simulink model "HW4_2a_gradient_discrete_time_proj_bad"  (R2023b)
settings: Solver=VariableStepAuto  StartTime=0.0  StopTime=700  RelTol=1e-3
model workspace (MAT data in the model file):
  M = Simulink.Parameter
  M.Value = 0.5
  M.DataType = 'auto'
  M.Complexity = 'real'
  M.Dimensions = [1 1]
  alpha = Simulink.Parameter
  alpha.Value = 1
  alpha.DataType = 'auto'
  alpha.Complexity = 'real'
  alpha.Dimensions = [1 1]
  b = Simulink.Parameter
  b.Value = 0.1
  b.DataType = 'auto'
  b.Complexity = 'real'
  b.Dimensions = [1 1]
  k = Simulink.Parameter
  k.Value = 5
  k.DataType = 'auto'
  k.Complexity = 'real'
  k.Dimensions = [1 1]
  m = Simulink.Parameter
  m.Value = 20
  m.DataType = 'auto'
  m.Complexity = 'real'
  m.Dimensions = [1 1]
  minv = Simulink.Parameter
  minv.Value = 1
  minv.Description = 'This is written by the parameter writer block.
    | Unfortunately it needs a placeholder value, so just choosing that as 1.'
  minv.DataType = 'auto'
  minv.Complexity = 'real'
  minv.Dimensions = [1 1]
undefined symbols (not defined in the file): DiscIntNeverNeededParam
libraries: matrix_library x3
settings Model: Creator=kaleb  LastModifiedBy=kaleb

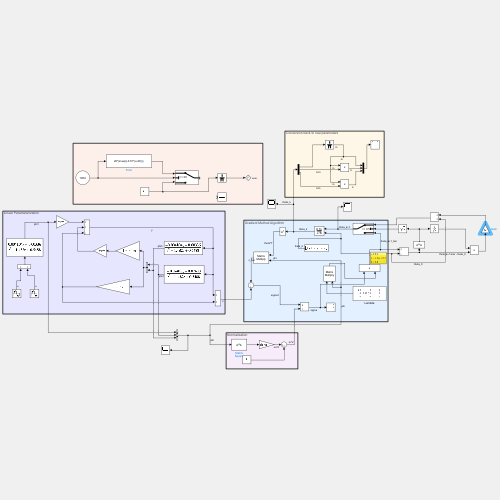
[thumbnail: Simulink's stored preview of the top-level diagram]
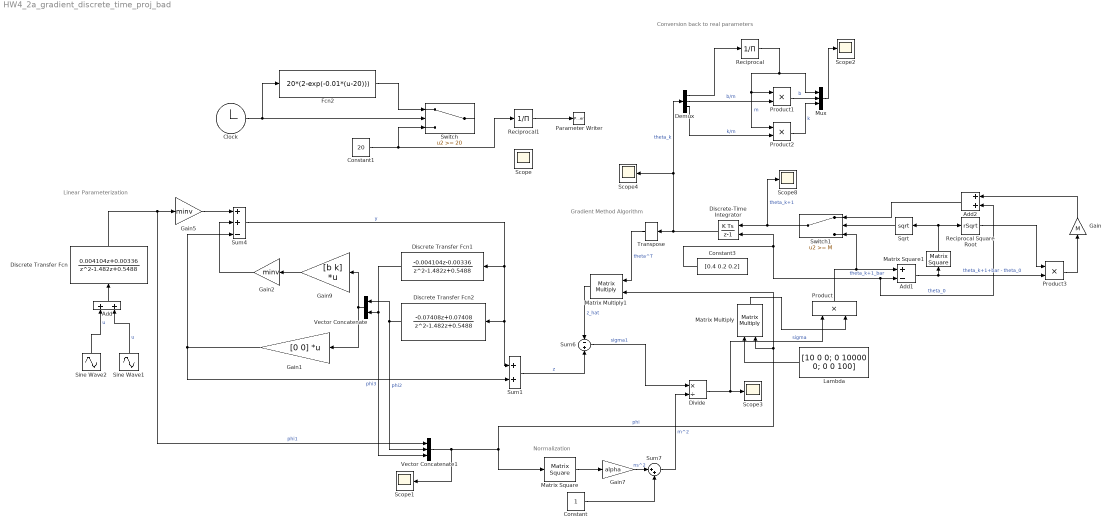
== system HW4_2a_gradient_discrete_time_proj_bad ==
  note: Gradient Method Algorithm
  note: Conversion back to real parameters
  note: Normalization
  note: Linear Parameterization
  Add : Sum
  Add1 : Sum  Inputs=+-
  Add2 : Sum
  Clock : Clock
  Constant : Constant
  Constant1 : Constant  Value=20
  Constant3 : Constant  Value=[0.4 0.2 0.2]
  Demux : Demux  Outputs=3
  Discrete Transfer Fcn : DiscreteTransferFcn  Numerator=[0.004104 0.00336]  Denominator=[1 -1.482 0.5488]
  Discrete Transfer Fcn1 : DiscreteTransferFcn  Numerator=[-0.004104 -0.00336]  Denominator=[1 -1.482 0.5488]
  Discrete Transfer Fcn2 : DiscreteTransferFcn  Numerator=[-0.07408 0.07408]  Denominator=[1 -1.482 0.5488]
  Discrete-Time Integrator : DiscreteIntegrator  InitialConditionSource=external  InitialCondition=[0.4 0.2 0.2]  SampleTime=-1  ICPrevOutput=DiscIntNeverNeededParam  ICPrevScaledInput=DiscIntNeverNeededParam
  Divide : Product  Inputs=*/
  Fcn2 : Fcn  Expr=20*(2-exp(-0.01*(u-20)))
  Gain : Gain  Gain=M
  Gain1 : Gain  Gain=[0 0]  Multiplication=Matrix(K*u)
  Gain2 : Gain  Gain=minv
  Gain5 : Gain  Gain=minv
  Gain7 : Gain  Gain=alpha
  Gain9 : Gain  Gain=[b k]  Multiplication=Matrix(K*u)
  Lambda : Constant  Value=[10 0 0; 0 10000 0; 0 0 100]
  Matrix Square : matrix_library/Matrix Square  OutMin=[]  OutMax=[]
      settings: LibrarySourceBlock=|
      | simulink/Matrix
      | Operations/Matrix
      | Square
  Matrix Square1 : matrix_library/Matrix Square  OutMin=[]  OutMax=[]
      settings: LibrarySourceBlock=|
      | simulink/Matrix
      | Operations/Matrix
      | Square
  Matrix Multiply : Product  Multiplication=Matrix(*)
  Matrix Multiply1 : Product  Multiplication=Matrix(*)
  Mux : Mux  Inputs=3
  Parameter Writer : ParameterWriter  AccessWorkspaceVariable=on  WorkspaceVariableName=minv
  Product{,1..3} (4 alike) : Product
  Reciprocal : Product  Inputs=/  OutMax=[10000]
  Reciprocal Square Root : Sqrt  Operator=rSqrt
  Reciprocal1 : Product  Inputs=/
  Scope{,1..4,8} (6 alike) : Scope
  Sine Wave1 : Sin  Amplitude=5  Frequency=0.5  SampleTime=0.1
  Sine Wave2 : Sin  Amplitude=2  Frequency=2  SampleTime=0.1
  Sqrt : Sqrt
  Sum1 : Sum
  Sum4 : Sum  Inputs=++-
  Sum6 : Sum  Inputs=-+
  Sum7 : Sum  Inputs=|++
  Switch : Switch  Threshold=20  ZeroCross=off  SaturateOnIntegerOverflow=off  InputSameDT=off
  Switch1 : Switch  Threshold=M  SaturateOnIntegerOverflow=off  InputSameDT=off
  Transpose : matrix_library/Transpose
  Vector Concatenate : Concatenate
  Vector Concatenate1 : Concatenate  NumInputs=3
  wires:
  Discrete Transfer Fcn/1 -> Vector Concatenate1/1, Gain5/1  "phi1"
  Sum4/1 -> Discrete Transfer Fcn1/1, Sum1/1, Discrete Transfer Fcn2/1  "y"
  Discrete Transfer Fcn2/1 -> Vector Concatenate1/2, Vector Concatenate/1  "phi2"
  Gain9/1 -> Gain2/1
  Vector Concatenate1/1 -> Scope1/1, Matrix Multiply1/2, Matrix Multiply/2, Matrix Square/1  "phi"
  Matrix Multiply1/1 -> Sum6/1  "z_hat"
  Matrix Square/1 -> Gain7/1
  Constant/1 -> Sum7/2
  Sum7/1 -> Divide/2  "m^2"
  Gain7/1 -> Sum7/1  "ns^2"
  Sum6/1 -> Divide/1  "sigma1"
  Discrete-Time Integrator/1 -> Transpose/1, Demux/1, Scope4/1  "theta_k"
  Transpose/1 -> Matrix Multiply1/1  "theta^T"
  Divide/1 -> Scope3/1, Product/1  "sigma"
  Demux/2 -> Product1/2  "b/m"
  Demux/3 -> Product2/2  "k/m"
  Reciprocal/1 -> Product1/1, Product2/1, Mux/1  "m"
  Product1/1 -> Mux/2  "b"
  Product2/1 -> Mux/3  "k"
  Mux/1 -> Scope2/1
  Matrix Multiply/1 -> Product/2
  Gain5/1 -> Sum4/1
  Demux/1 -> Reciprocal/1
  Vector Concatenate/1 -> Gain9/1, Gain1/1
  Gain1/1 -> Sum4/3, Sum1/2
  Sum1/1 -> Sum6/2  "z"
  Lambda/1 -> Matrix Multiply/1
  Fcn2/1 -> Switch/1
  Clock/1 -> Fcn2/1, Switch/2
  Constant1/1 -> Reciprocal1/1, Switch/3
  Gain2/1 -> Sum4/2
  Sine Wave1/1 -> Add/2  "u"
  Discrete Transfer Fcn1/1 -> Vector Concatenate/2, Vector Concatenate1/3  "phi3"
  Reciprocal1/1 -> Parameter Writer/1
  Sine Wave2/1 -> Add/1  "u"
  Add/1 -> Discrete Transfer Fcn/1
  Constant3/1 -> Discrete-Time Integrator/2, Add2/2, Add1/2  "theta_0"
  Product/1 -> Switch1/3, Add1/1  "theta_k+1_bar"
  Switch1/1 -> Scope8/1, Discrete-Time Integrator/1  "theta_k+1"
  Add1/1 -> Product3/2, Matrix Square1/1  "theta_k+1+bar - theta_0"
  Product3/1 -> Gain/1
  Reciprocal Square Root/1 -> Product3/1
  Gain/1 -> Add2/1
  Add2/1 -> Switch1/1
  Matrix Square1/1 -> Reciprocal Square Root/1, Sqrt/1
  Sqrt/1 -> Switch1/2
